simulink model "Pendulum_dynamics_2021a"  (R2021a)
settings: Solver=FixedStepAuto  StartTime=0  StopTime=t_final  FixedStep=t_step  MaxStep=t_step  MinStep=t_step  RelTol=1e-3  AbsTol=0
values from neighbouring files (symbols this model uses):
  b = 5    [Task1_ILC_.m]    (also in Task2_ILC_FF_.m)
  g = 9.81    [Motion_control.m]    (also in RPRP_dynamics_with_spring.m; Task1_ILC_.m; Task2_ILC_FF_.m; ode_solver_full_spring.m)
  l = 1    [Task1_ILC_.m]    (also in Task2_ILC_FF_.m)
  m = 2    [Task1_ILC_.m]    (also in Task2_ILC_FF_.m)
settings Model: Creator=admin  LastModifiedBy=Ashut
settings SolverCC: InitialStep=t_step
settings DebuggingCC: UnconnectedInputMsg=none  UnconnectedOutputMsg=none  UnconnectedLineMsg=none
settings ModelReferenceCC: EnableRefExpFcnMdlSchedulingChecks=off
settings RTWCC: Description=Generic Real-Time Target  DLArmComputeVersion=20.02.1

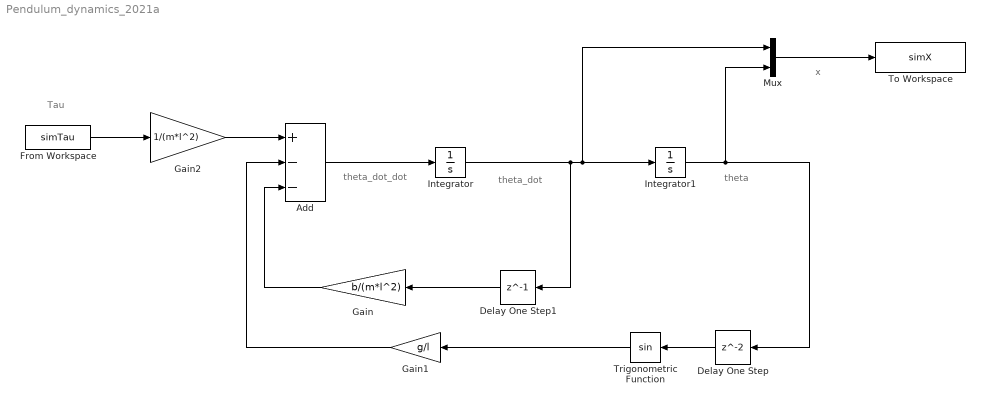
== system Pendulum_dynamics_2021a ==
  note: x
  note: Tau
  note: theta
  note: theta_dot
  note: theta_dot_dot
  Add : Sum  Inputs=+--
  Delay One Step : Delay
  Delay One Step1 : Delay  DelayLength=1
  From Workspace : FromWorkspace  VariableName=simTau
  Gain : Gain  Gain=b/(m*l^2)
  Gain1 : Gain  Gain=g/l
  Gain2 : Gain  Gain=1/(m*l^2)
  Integrator : Integrator
  Integrator1 : Integrator
  Mux : Mux  Inputs=2
  To Workspace : ToWorkspace  VariableName=simX  SaveFormat=Timeseries  SampleTime=-1
  Trigonometric Function : Trigonometry
  wires:
  Add/1 -> Integrator/1
  Gain2/1 -> Add/1
  Gain/1 -> Add/3
  Gain1/1 -> Add/2
  Trigonometric Function/1 -> Gain1/1
  Integrator1/1 -> Mux/2, Delay One Step/1
  Integrator/1 -> Delay One Step1/1, Mux/1, Integrator1/1
  From Workspace/1 -> Gain2/1
  Mux/1 -> To Workspace/1
  Delay One Step/1 -> Trigonometric Function/1
  Delay One Step1/1 -> Gain/1
